simulink model "client_dspassign1"  (R2018b)
settings: Solver=FixedStepDiscrete  StartTime=0.0  StopTime=inf  RelTol=1e-3
undefined symbols (not defined in the file): Button, unt_c
libraries: androidaudiovideolib x5, dspfdesign x2, androidcommunicationlib x2, androiduilib x1
settings Model: Creator=gajen  LastModifiedBy=gajen
settings OptimizationCC: EnhancedBackFolding=on  PassReuseOutputArgsAs=Individual arguments  MaxStackSize=64  OptimizeBlockOrder=speed  DifferentSizesBufferReuse=on  OptimizationCustomize=off
settings DebuggingCC: ParameterTunabilityLossMsg=error
settings HardwareCC: ProdBitPerPointer=32  ProdBitPerSizeT=32  ProdBitPerPtrDiffT=32  ProdLargestAtomicInteger=Long  ProdLargestAtomicFloat=Double  ProdWordSize=32  ProdHWDeviceType=ARM Compatible->ARM Cortex
settings SFSimCC: MATLABDynamicMemAlloc=off
settings RTWCC: SystemTargetFile=ert.tlc  HardwareBoard=Android Device  TLCOptions="-aInlineSetEventsForThisBaseRateFcn=TLC_FALSE -aSuppressMultiTaskScheduler=TLC_FALSE  -aRateBasedStepFcn=0"  TemplateMakefile=ert_default_tmf  GenerateReport=on  RTWVerbose=off  Toolchain=Android SDK/NDK Tools  BuildConfiguration=Faster Runs  IncludeHyperlinkInReport=on  LaunchReport=on  GenerateTraceInfo=on  GenerateTraceReport=on  GenerateTraceReportSl=on  GenerateTraceReportSf=on  GenerateTraceReportEml=on
settings CodeAppCC: ForceParamTrailComments=on  IgnoreCustomStorageClasses=off  OperatorAnnotations=on  SimulinkDataObjDesc=on  SFDataObjDesc=on  InsertBlockDesc=on

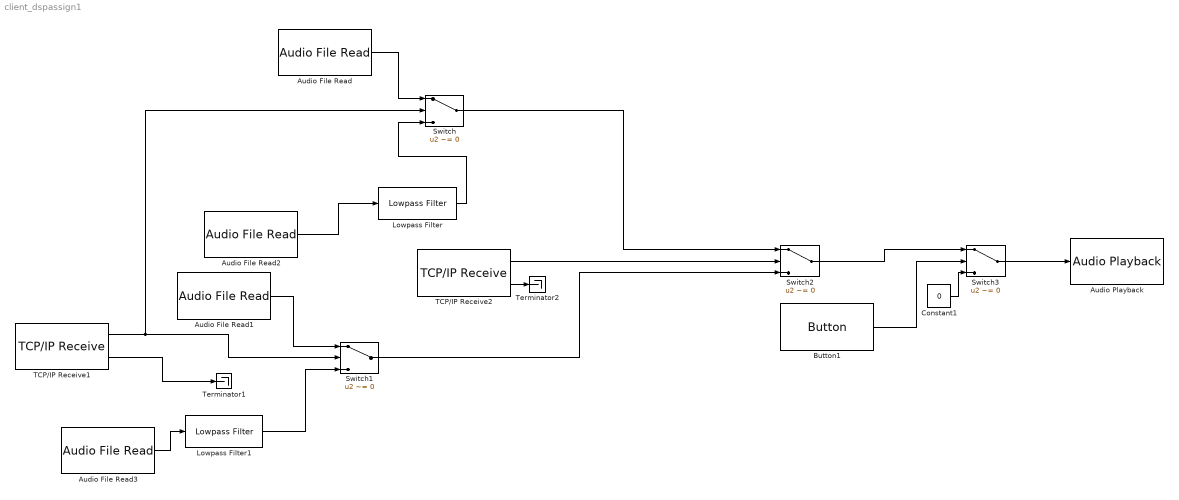
== system client_dspassign1 ==
  Audio File Read : androidaudiovideolib/Audio File Read  FileName=C:\Users\gajen\OneDrive\Desktop\music\Mere Sapno Ki Rani - Aradhana - Rajesh Khanna & Sharmila Tagore - Superhit Song.mp3  FrameSize=4410
      settings: SourceProductName=Simulink Support Package for Android Devices  SourceProductBaseCode=ANDROID
  Audio File Read1 : androidaudiovideolib/Audio File Read  FileName=C:\Users\gajen\OneDrive\Desktop\music\Zindagi Ke Safar Mein Guzar Jaate Kishore Kumar Aap Ki Kasam 1974 Songs.mp3  FrameSize=4410
      settings: SourceProductName=Simulink Support Package for Android Devices  SourceProductBaseCode=ANDROID
  Audio File Read2 : androidaudiovideolib/Audio File Read  FileName=C:\Users\gajen\OneDrive\Desktop\music\Mere Sapno Ki Rani - Aradhana - Rajesh Khanna & Sharmila Tagore - Superhit Song.mp3  FrameSize=4410
      settings: SourceProductName=Simulink Support Package for Android Devices  SourceProductBaseCode=ANDROID
  Audio File Read3 : androidaudiovideolib/Audio File Read  FileName=C:\Users\gajen\OneDrive\Desktop\music\Zindagi Ke Safar Mein Guzar Jaate Kishore Kumar Aap Ki Kasam 1974 Songs.mp3  FrameSize=4410
      settings: SourceProductName=Simulink Support Package for Android Devices  SourceProductBaseCode=ANDROID
  Audio Playback : androidaudiovideolib/Audio Playback  SampleFreq=44100  AudioSamplingFreq=44100  SampleTime=0.1  DeviceStr=0  QueueDuration=0  BlockPlatform=Android
      settings: SourceProductName=Simulink Support Package for Android Devices  SourceProductBaseCode=ANDROID
  Button1 : androiduilib/Button  ButtonState=Not pressed  ButtonId=unt_c/Button  State=off  SampleTime=0.1  BlockPlatform=Android
      settings: SourceProductName=Simulink Support Package for Android Devices  SourceProductBaseCode=ANDROID
  Constant1 : Constant  Value=0
  Lowpass Filter : dspfdesign/Lowpass Filter  FilterType=FIR  DesignForMinimumOrder=on  FilterOrder=50  PassbandFrequency=1  StopbandFrequency=1e3  PassbandRipple=0.0001  StopbandAttenuation=40  InheritSampleRate=off  SampleRate=44100  SimulateUsing=Interpreted execution  roundingMode=Floor  coeffsDataTypeStr=fixdt(1,16)
  Lowpass Filter1 : dspfdesign/Lowpass Filter  FilterType=FIR  DesignForMinimumOrder=on  FilterOrder=50  PassbandFrequency=1  StopbandFrequency=1e3  PassbandRipple=0.0001  StopbandAttenuation=40  InheritSampleRate=off  SampleRate=44100  SimulateUsing=Interpreted execution  roundingMode=Floor  coeffsDataTypeStr=fixdt(1,16)
  Switch{,1..3} (4 alike) : Switch  Criteria=u2 ~= 0
  TCP/IP Receive1 : androidcommunicationlib/TCP//IP Receive  TCPReceiveId=unt_c/TCP//IP_Receive1  Mode_=Client  LocalServerPort_=25000  RemoteAddr_=10.1.131.205  RemoteServerPort_=25001  DataType_=boolean  DataSize_=1  SampleTime_=0.1  SimulateUsing=Code generation  ClientPortBindingSelection_=off  ClientPortToBind_=35000  BlockingMode_=off  BlockTimeout_=0.1
      settings: SourceProductName=Simulink Support Package for Android Devices  SourceProductBaseCode=ANDROID
  TCP/IP Receive2 : androidcommunicationlib/TCP//IP Receive  TCPReceiveId=unt_c/TCP//IP_Receive1  Mode_=Client  LocalServerPort_=25000  RemoteAddr_=10.1.131.205  RemoteServerPort_=25002  DataType_=boolean  DataSize_=1  SampleTime_=0.1  SimulateUsing=Code generation  ClientPortBindingSelection_=off  ClientPortToBind_=35000  BlockingMode_=off  BlockTimeout_=0.1
      settings: SourceProductName=Simulink Support Package for Android Devices  SourceProductBaseCode=ANDROID
  Terminator1 : Terminator
  Terminator2 : Terminator
  wires:
  Audio File Read/1 -> Switch/1
  TCP/IP Receive1/1 -> Switch/2, Switch1/2
  Audio File Read1/1 -> Switch1/1
  Lowpass Filter/1 -> Switch/3
  Audio File Read2/1 -> Lowpass Filter/1
  Audio File Read3/1 -> Lowpass Filter1/1
  Switch/1 -> Switch2/1
  Switch1/1 -> Switch2/3
  TCP/IP Receive2/1 -> Switch2/2
  Lowpass Filter1/1 -> Switch1/3
  TCP/IP Receive1/2 -> Terminator1/1
  Switch3/1 -> Audio Playback/1
  Switch2/1 -> Switch3/1
  Button1/1 -> Switch3/2
  Constant1/1 -> Switch3/3
  TCP/IP Receive2/2 -> Terminator2/1
